simulink model "Continuous_Dc_Motor_Model"  (R2024a)
settings: Solver=ode23s  StartTime=0.0  StopTime=10.0
model workspace (MAT data in the model file):
  J = 5e-05
  K = 0.2
  L = 0.01
  R = 4
  Ts = 0.01
  V = 7.4
  a1 = 0.5
  a2 = 2
  a3 = 2.5
  b = 5e-05
  ki = 7.33
  kp = 9.39
settings Model: Creator=BIDO  LastModifiedBy=BIDO

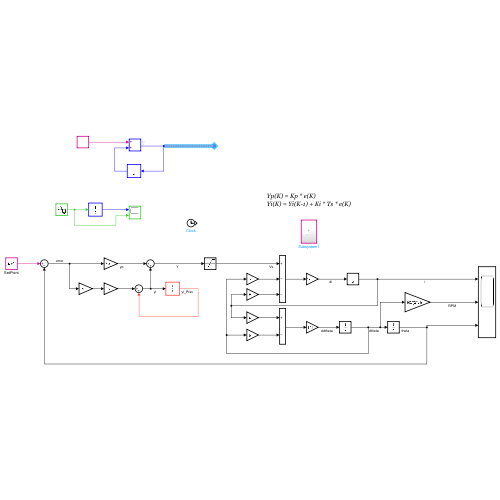
[thumbnail: Simulink's stored preview of the top-level diagram]
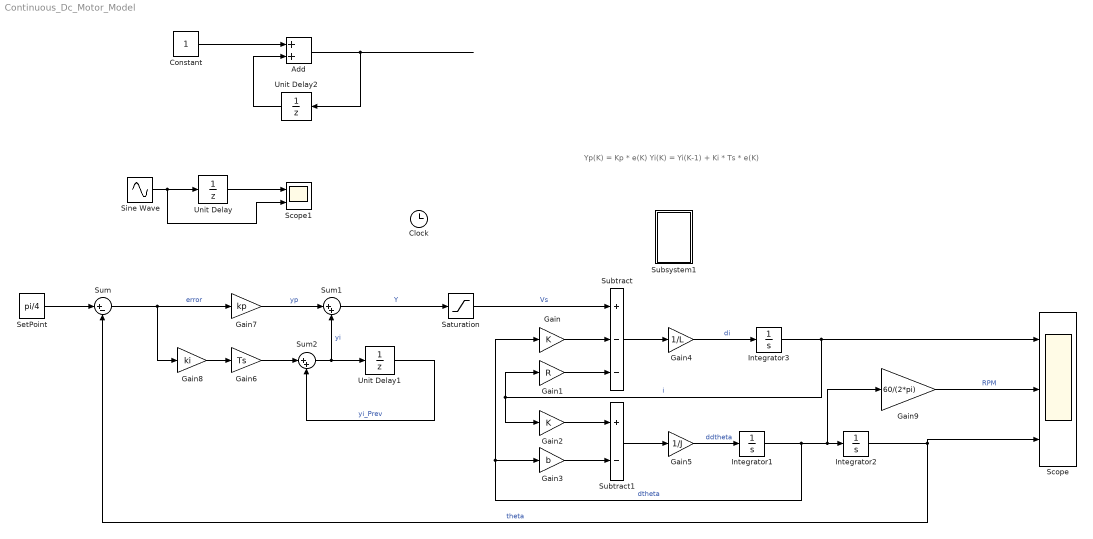
== system Continuous_Dc_Motor_Model ==
  note: Yp(K) = Kp * e(K)
      | Yi(K) = Yi(K-1) + Ki * Ts * e(K)
  Add : Sum
  Clock : Clock
  Constant : Constant
  Gain : Gain  Gain=K
  Gain1 : Gain  Gain=R
  Gain2 : Gain  Gain=K
  Gain3 : Gain  Gain=b
  Gain4 : Gain  Gain=1/L
  Gain5 : Gain  Gain=1/J
  Gain6 : Gain  Gain=Ts
  Gain7 : Gain  Gain=kp
  Gain8 : Gain  Gain=ki
  Gain9 : Gain  Gain=60/(2*pi)
  Integrator1 : Integrator  ContinuousStateAttributes='Velocity'
  Integrator2 : Integrator  ZeroCross=off  ContinuousStateAttributes='Angle'
  Integrator3 : Integrator
  Saturation : Saturate  UpperLimit=V  LowerLimit=-V
  Scope : Scope  NumInputPorts=3
  Scope1 : Scope  NumInputPorts=2
  SetPoint : Constant  Value=pi/4
  Sine Wave : Sin  Phase=pi/2  SampleTime=0.4
  Subsystem1 : Subsystem
  Subtract : Sum  Inputs=+--
  Subtract1 : Sum  Inputs=+-
  Sum : Sum  Inputs=|+-
  Sum1 : Sum  Inputs=|++
  Sum2 : Sum  Inputs=|++
  Unit Delay : UnitDelay  SampleTime=0.8  HasFrameUpgradeWarning=on
  Unit Delay1 : UnitDelay  SampleTime=Ts  HasFrameUpgradeWarning=on
  Unit Delay2 : UnitDelay  HasFrameUpgradeWarning=on
  wires:
  Sum1/1 -> Saturation/1  "Y"
  Gain1/1 -> Subtract/3
  Gain/1 -> Subtract/2
  Gain2/1 -> Subtract1/1
  Gain3/1 -> Subtract1/2
  Integrator3/1 -> Gain1/1, Gain2/1, Scope/1  "i"
  Subtract/1 -> Gain4/1
  Gain4/1 -> Integrator3/1  "di"
  Subtract1/1 -> Gain5/1
  Gain5/1 -> Integrator1/1  "ddtheta"
  Integrator1/1 -> Gain3/1, Gain/1, Gain9/1, Integrator2/1  "dtheta"
  Sum/1 -> Gain8/1, Gain7/1  "error"
  Gain7/1 -> Sum1/1  "yp"
  Gain8/1 -> Gain6/1
  Gain6/1 -> Sum2/1
  Sum2/1 -> Sum1/2, Unit Delay1/1  "yi"
  Integrator2/1 -> Sum/2, Scope/3  "theta"
  Unit Delay1/1 -> Sum2/2  "yi_Prev"
  Gain9/1 -> Scope/2  "RPM"
  Saturation/1 -> Subtract/1  "Vs"
  SetPoint/1 -> Sum/1
  Sine Wave/1 -> Unit Delay/1, Scope1/2
  Unit Delay/1 -> Scope1/1
  Constant/1 -> Add/1
  Add/1 -> Unit Delay2/1
  Unit Delay2/1 -> Add/2

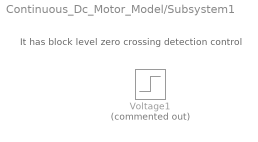
== system Continuous_Dc_Motor_Model/Subsystem1 ==
  note: It has block level zero crossing detection control
  Voltage1 : Step  Commented=on  After=V  SampleTime=0
